simulink model "controlefourv2"  (R2021a)
settings: Solver=ode15s  StartTime=0.0  StopTime=400.0  FixedStep=0.1  RelTol=1e-3  EnableMultiTasking=on
settings Model: NumberOfSteps=10  Creator=M1  LastModifiedBy=M1
settings SolverCC: AlgebraicLoopSolver=TrustRegion  AutoInsertRateTranBlk=on
settings DataIOCC: LimitDataPoints=on  ReturnWorkspaceOutputs=off
settings OptimizationCC: LifeSpan=inf
settings DebuggingCC: AllowSymbolicDim=off  SFUnexpectedBacktrackingDiag=warning  SFNoUnconditionalDefaultTransitionDiag=warning  SFExecutionAtInitializationDiag=none  SFMachineParentedDataDiag=warning  ArithmeticOperatorsInVariantConditions=warning
settings SFSimCC: SimUseLocalCustomCode=off  CustomCodeUndefinedFunction=UseInterfaceOnly
settings RTWCC: RTWUseLocalCustomCode=off
settings CodeAppCC: StateflowObjectComments=on
settings GRTTargetCC: TargetLangStandard=C89/C90 (ANSI)
settings ConfigComp: CovMetricSettings=dw  CovSaveCumulativeToWorkspaceVar=on  CovSaveSingleToWorkspaceVar=on  CovExternalEMLEnable=off  CovSFcnEnable=off

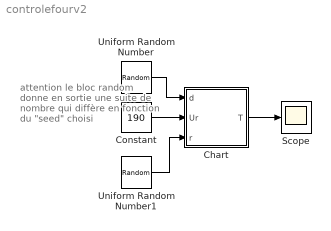
== system controlefourv2 ==
  note: attention
      | le bloc random
      | donne en sortie
      | une suite de nombre
      | qui diffère en fonction
      | du "seed" choisi
  Chart : Stateflow chart  TreatAsAtomicUnit=on
  Constant : Constant  Value=190
  Scope : Scope
  Uniform Random Number : UniformRandomNumber  Minimum=0  Seed=1  SampleTime=40
  Uniform Random Number1 : UniformRandomNumber  Minimum=0  SampleTime=5
  wires:
  Chart/1(T) -> Scope/1
  Constant/1 -> Chart/2(Ur)
  Uniform Random Number/1 -> Chart/1(d)
  Uniform Random Number1/1 -> Chart/3(r)

== stateflow chart controlefourv2/Chart ==
  settings: updateMethod=CONTINUOUS
  note: Rien ne corrige le four en panne
      | à cet état
  state normal
    during :
    T_dot = -0.15*T +0.15*Ur;
  state PIdef
    during :
    T_dot = -1/15*T + 1/15*Umax;
  note: Umin et Umax sont les tempéraure que risquent atteindre le
      | four une fois qu'il est suprevisé par le sous correcteur.
      | Tinf et Tsup sont les bornes que l'on souhaite limiter les four
      | lorsqu'il y a une panne
  note: On assume que le four reste impeccable après réparation
      | le temps qu'il atteigne la température souhaité
  state PIpanne
    state TORactive
      state TORmax
        during :
        T_dot = -1/15*T + 1/15*Umin;
      state TORmin
        during :
        T_dot = -1/15*T + 1/15*Umax;
      TORmin -> TORmax : [T>Tsup]
      TORmax -> TORmin : [T<Tinf]
    state TORdef
      during :
      T_dot = -1/15*T + 1/15*Umin;
    note: Les deux correcteurs est en panne
    TORdef -> TORmax : [after(10, sec)]
    TORactive -> TORdef : [r < 0.05]
  state repare
    during :
    T_dot = -0.15*T +0.15*Ur;
  note: La température s'éloigne de la borne sup
  note: La température s'éloigne de la borne inf
  (default) -> normal
  normal -> PIdef : [d < 0.1]
  PIdef -> TORmax : [after(0.1, sec) && T > Tmax]
  repare -> normal : [abs(T - Ur) < 0.1]
  PIpanne -> repare : [after(40,sec)]
  data: T output =25; d input; Ur input; Umax constant double =300; Umin constant double =0; Tmax constant double =240; Tinf constant double =170; Tsup constant double =210; r input
  data T settings: updateMethod=SF_CONTINUOUS_TIME_DATA
